simulink library "formationFlyingBlockset"  (R2016b)
settings: Solver=ode45  StartTime=0.0  StopTime=10.0  RelTol=1e-3  EnableMultiTasking=on
undefined symbols (not defined in the file or in its folder): adaptive, aircraftmask_ID, aircraftmask_navigationLaw, aircraftmask_originNED_ECEF_rrm, aircraftmask_p0_NED_m, aircraftmask_phithetapsi_trim, aircraftmask_wakevortexenabled, airkraftmask_displayLeader, DiscIntNeverNeededParam, Earth, fflib_degdegm2rrm, fflib_Hz2radps, fflib_rrm2degdegm, flat2lla, hinf, Klqr, lquadr, mask_ac, mask_ID, mpc, poleplacement, uavsim, washout, WGS84
undefined symbols (not defined in the file): aircraftmask_phithetapsi0, aircraftmask_pqr0, aircraftmask_uvw0, innerloop, outerloop, tatestos
libraries: formationFlyingBlockset x59, aerolibtransform2 x42, simulink_extras x27, dspsrcs4 x11, aerolibutil x5, uavsimBlockset_UAV3DInterface x4, uavsimBlockset_ServoHS55 x4, uavsimBlockset_VectorNorm x3, uavsimBlockset_UAV3DVisualization x3, uavsimBlockset_AugmentWind x3, stringquartett x2, Parrot_DCAS_lib x2
(part 5 of 5)

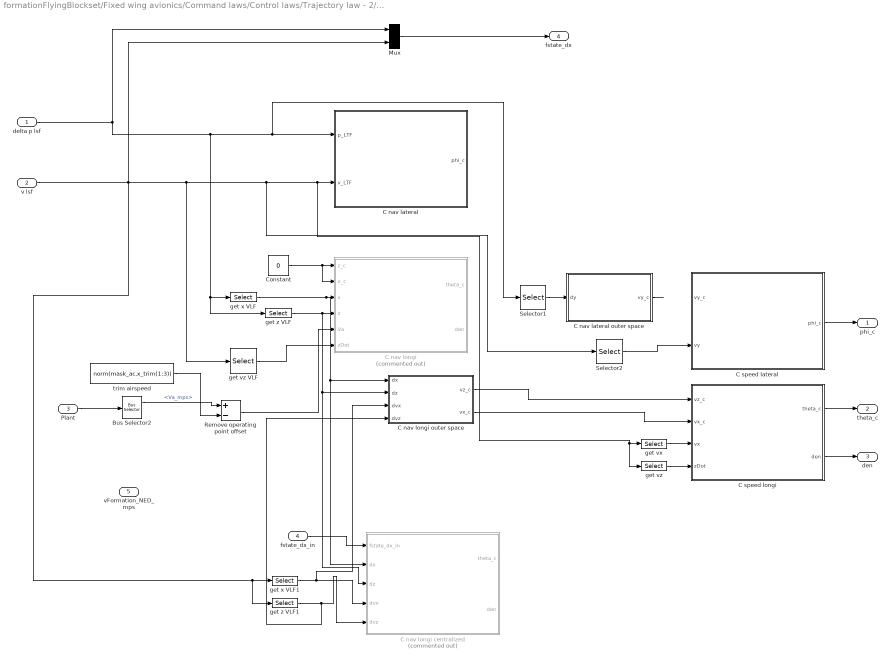
== system formationFlyingBlockset/Fixed wing avionics/Command laws/Control laws/Trajectory law - 2/Leader following laws/LQR nav loops ==
  delta p lsf : Inport
  v lsf : Inport  Port=2
  Plant : Inport  Port=3  OutDataTypeStr=Bus: StateBus
  fstate_dx_in : Inport  Port=4
  vFormation_NED_mps : Inport  Port=5
  Bus Selector2 : BusSelector  OutputSignals=Va_mps,v_ned_mps
  C nav lateral : Subsystem
  C nav lateral outer space : Subsystem
  C nav longi : Subsystem  Commented=on
  C nav longi centralized : Subsystem  Commented=on
  C nav longi outer space : Subsystem
  C speed lateral : Subsystem
  C speed longi : Subsystem
  Constant : Constant  Value=0
  Mux : Mux  Inputs=2
  Remove operating point offset : Sum  Inputs=+-
  Selector1 : Selector  InputPortWidth=3  IndexOptions=Index vector (dialog)  Indices=2  OutputSizes=1
  Selector2 : Selector  InputPortWidth=3  IndexOptions=Index vector (dialog)  Indices=2  OutputSizes=1
  get vx : Selector  InputPortWidth=3  IndexOptions=Index vector (dialog)  Indices=1  OutputSizes=1
  get vz : Selector  InputPortWidth=3  IndexOptions=Index vector (dialog)  Indices=3  OutputSizes=1
  get vz VLF : Selector  InputPortWidth=3  IndexOptions=Index vector (dialog)  Indices=3  OutputSizes=1
  get x VLF : Selector  InputPortWidth=3  IndexOptions=Index vector (dialog)  Indices=1  OutputSizes=1
  get x VLF1 : Selector  InputPortWidth=3  IndexOptions=Index vector (dialog)  Indices=1  OutputSizes=1
  get z VLF : Selector  InputPortWidth=3  IndexOptions=Index vector (dialog)  Indices=3  OutputSizes=1
  get z VLF1 : Selector  InputPortWidth=3  IndexOptions=Index vector (dialog)  Indices=3  OutputSizes=1
  trim airspeed : Constant  Value=norm(mask_ac.x_trim(1:3))
  phi_c : Outport  PortDimensions=1
  theta_c : Outport  Port=2  PortDimensions=1
  den : Outport  Port=3  PortDimensions=1
  fstate_dx : Outport  Port=4
  wires:
  C speed lateral/1(phi_c) -> phi_c/1
  v lsf/1 -> Mux/2, get vz VLF/1, C nav lateral/2(v_LTF), get vx/1, get vz/1, Selector2/1, get x VLF1/1, get z VLF1/1
  Selector2/1 -> C speed lateral/2(vy)
  C nav lateral outer space/1(vy_c) -> ?
  Selector1/1 -> C nav lateral outer space/1(dy)
  get z VLF1/1 -> C nav longi centralized/5(dvz), C nav longi outer space/4(dvz)
  C nav longi outer space/2(vx_c) -> C speed longi/2(vx_c)
  C nav longi outer space/1(vz_c) -> C speed longi/1(vz_c)
  get vz/1 -> C speed longi/4(zDot)
  get vx/1 -> C speed longi/3(vx)
  get x VLF1/1 -> C nav longi centralized/4(dvx), C nav longi outer space/3(dvx)
  delta p lsf/1 -> Mux/1, get z VLF/1, get x VLF/1, C nav lateral/1(p_LTF), Selector1/1
  Constant/1 -> C nav longi/2(x_c), C nav longi/1(z_c)
  get z VLF/1 -> C nav longi/4(z), C nav longi centralized/3(dz), C nav longi outer space/2(dz)
  get x VLF/1 -> C nav longi/3(x), C nav longi centralized/2(dx), C nav longi outer space/1(dx)
  Remove operating point offset/1 -> C nav longi/5(Va)
  get vz VLF/1 -> C nav longi/6(zDot)
  C speed longi/1(theta_c) -> theta_c/1
  C speed longi/2(den) -> den/1
  Plant/1 -> Bus Selector2/1
  Bus Selector2/1 -> Remove operating point offset/1  "<Va_mps>"
  trim airspeed/1 -> Remove operating point offset/2
  fstate_dx_in/1 -> C nav longi centralized/1(fstate_dx_in)
  Mux/1 -> fstate_dx/1

== system formationFlyingBlockset/Fixed wing avionics/Command laws/Control laws/Trajectory law - 2/Leader following laws/Manual tuning SISO outer loops ==
  "\tIntegrator reset signal" : Inport
  v lsf : Inport  Port=2
  p lsf : Inport  Port=3
  Trigger : TriggerPort  TriggerType=either  VariantControl=Variant  PortDimensions=1
  Altitude controller : Subsystem
  Lateral trajectory deviation controller : Subsystem
  Longitudinal trajectory deviation controller : Subsystem
  theta_c : Outport
  phi_c : Outport  Port=2
  delta_en : Outport  Port=3
  wires:
  Altitude controller/1(theta_c) -> theta_c/1
  "\tIntegrator reset signal"/1 -> Longitudinal trajectory deviation controller/3(Integrator Reset), Altitude controller/1(Integrator Reset)
  Longitudinal trajectory deviation controller/1(delta_en) -> delta_en/1
  Lateral trajectory deviation controller/1(phi_c) -> phi_c/1
  p lsf/1 -> Altitude controller/3(p lsf), Longitudinal trajectory deviation controller/1(p_ERRF), Lateral trajectory deviation controller/1(p_ERRF)
  v lsf/1 -> Lateral trajectory deviation controller/2(v_ERRF), Altitude controller/2(v lsf), Longitudinal trajectory deviation controller/2(v_ERRF)

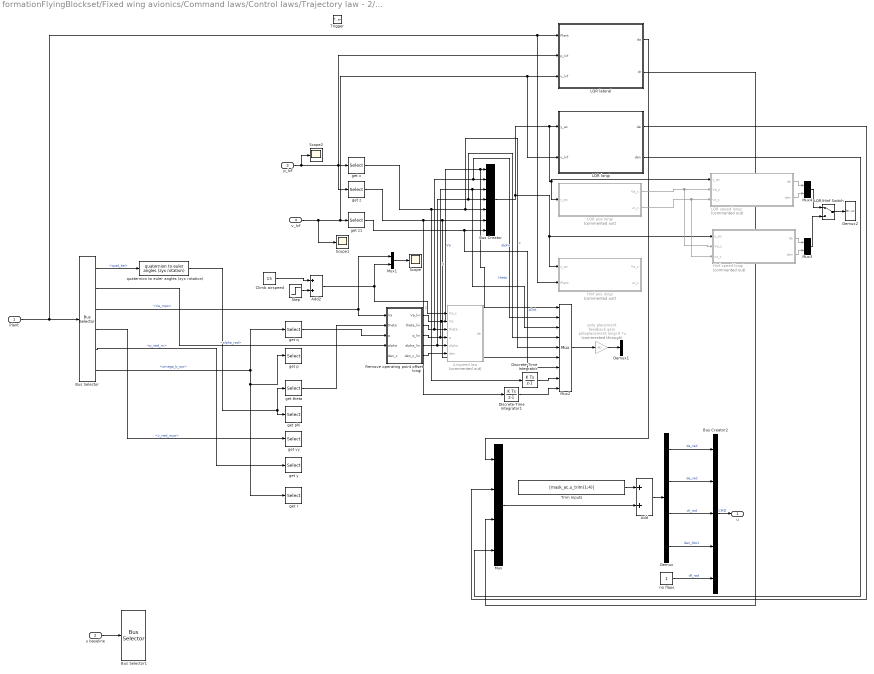
== system formationFlyingBlockset/Fixed wing avionics/Command laws/Control laws/Trajectory law - 2/Leader following laws/Non-nested laws ==
  Plant : Inport  OutDataTypeStr=Bus: StateBus
  u baseline : Inport  Port=2  OutDataTypeStr=Bus: CMD
  p_lvf : Inport  Port=3
  v_lvf : Inport  Port=4
  Trigger : TriggerPort  TriggerType=either  VariantControl=Variant  PortDimensions=1
  Add : Sum
  Add2 : Sum
  Airspeed law : Subsystem  Commented=on
  Bus Creator : BusCreator  Inputs='Va','theta','q','alpha','x','z','zDot'
  Bus Creator2 : BusCreator  Inputs=5  OutDataTypeStr=Bus: CMD  NonVirtualBus=on
  Bus Selector : BusSelector  OutputSignals=quat_be,alpha_rad,Va_mps,v_ned_mps,p_ned_m,omega_b_rps
  Bus Selector1 : BusSelector  OutputSignals=da_rad,de_rad,den_0to1
  Climb airspeed : Constant  Value=15
  Demux : Demux
  Demux1 : Demux  Outputs=2
  Demux2 : Demux  Outputs=2
  Discrete-Time Integrator : DiscreteIntegrator  InitialConditionSetting=State (most efficient)  SampleTime=-1  ICPrevOutput=DiscIntNeverNeededParam  ICPrevScaledInput=DiscIntNeverNeededParam
  Discrete-Time Integrator1 : DiscreteIntegrator  InitialConditionSetting=State (most efficient)  SampleTime=-1  ICPrevOutput=DiscIntNeverNeededParam  ICPrevScaledInput=DiscIntNeverNeededParam
  Hinf pos longi : Subsystem  Commented=on
  Hinf speed longi : Subsystem  Commented=on
  LQR lateral : Subsystem
  LQR longi : Subsystem
  LQR pos longi : Subsystem  Commented=on
  LQR speed longi : Subsystem  Commented=on
  LQR/Hinf Switch : ManualSwitch
  Mux : Mux
  Mux1 : Mux  Inputs=2
  Mux2 : Mux  Inputs=9
  Mux3 : Mux  Inputs=2
  Mux4 : Mux  Inputs=2
  Remove operating point offset longi : Subsystem
  Scope : Scope
  Scope1 : Scope
  Scope2 : Scope
  Step : Step  Time=12  After=5
  Trim Inputs : Constant  Value=[mask_ac.u_trim(1:4)]
  get p : Selector  InputPortWidth=3  IndexOptions=Index vector (dialog)  Indices=[1]  OutputSizes=1
  get phi : Selector  InputPortWidth=3  IndexOptions=Index vector (dialog)  Indices=[1]  OutputSizes=1
  get q : Selector  InputPortWidth=3  IndexOptions=Index vector (dialog)  Indices=2  OutputSizes=1
  get r : Selector  InputPortWidth=3  IndexOptions=Index vector (dialog)  Indices=3  OutputSizes=1
  get theta : Selector  InputPortWidth=3  IndexOptions=Index vector (dialog)  Indices=2  OutputSizes=1
  get vy : Selector  InputPortWidth=3  IndexOptions=Index vector (dialog)  Indices=2  OutputSizes=1
  get x : Selector  InputPortWidth=3  IndexOptions=Index vector (dialog)  Indices=1  OutputSizes=1
  get y : Selector  InputPortWidth=3  IndexOptions=Index vector (dialog)  Indices=2  OutputSizes=1
  get z : Selector  InputPortWidth=3  IndexOptions=Index vector (dialog)  Indices=3  OutputSizes=1
  get z1 : Selector  InputPortWidth=3  IndexOptions=Index vector (dialog)  Indices=3  OutputSizes=1
  no flaps : Constant
  pole placement feedback gain : Gain  Commented=through  Gain=poleplacement.longi.K  Multiplication=Matrix(K*u)
  quaternion to euler angles (zyx rotation) : formationFlyingBlockset/quaternion to euler  angles (zyx rotation)
  u : Outport  OutDataTypeStr=Bus: CMD
  wires:
  Bus Creator2/1 -> u/1  "CMD"
  Demux/3 -> Bus Creator2/3  "dr_rad"
  Demux/4 -> Bus Creator2/4  "den_0to1"
  Demux/1 -> Bus Creator2/1  "da_rad"
  Demux/2 -> Bus Creator2/2  "de_rad"
  Trim Inputs/1 -> Add/1
  Add/1 -> Demux/1
  Mux/1 -> Add/2
  no flaps/1 -> Bus Creator2/5  "df_rad"
  quaternion to euler angles (zyx rotation)/1 -> get phi/1, get theta/1
  Bus Selector/2 -> Remove operating point offset longi/4(alpha)  "<alpha_rad>"
  Bus Selector/3 -> Remove operating point offset longi/1(Va), Mux1/1  "<Va_mps>"
  Climb airspeed/1 -> Add2/1
  Step/1 -> Add2/2
  get theta/1 -> Remove operating point offset longi/2(theta)
  Bus Selector/4 -> get vy/1  "<v_ned_mps>"
  Bus Selector/5 -> get y/1  "<p_ned_m>"
  Bus Selector/6 -> get r/1, get p/1, get q/1  "<omega_b_rps>"
  get q/1 -> Remove operating point offset longi/3(q)
  u baseline/1 -> Bus Selector1/1
  Remove operating point offset longi/5(den_c_lin) -> Airspeed law/6(den)
  Add2/1 -> Airspeed law/1(Va_c), Mux1/2
  Mux1/1 -> Scope/1
  Bus Selector/1 -> quaternion to euler angles (zyx rotation)/1  "<quat_be>"
  Remove operating point offset longi/1(Va_lin) -> Mux2/1, Bus Creator/1, Airspeed law/2(Va)  "Va"
  get x/1 -> Discrete-Time Integrator/1, Mux2/5, Bus Creator/5  "x"
  get z/1 -> Discrete-Time Integrator1/1, Bus Creator/6, Mux2/6  "z"
  Remove operating point offset longi/2(theta_lin) -> Mux2/2, Bus Creator/2, Airspeed law/3(theta)  "theta"
  Remove operating point offset longi/3(q_lin) -> Mux2/3, Bus Creator/3, Airspeed law/4(q)  "q"
  Remove operating point offset longi/4(alpha_lin) -> Mux2/4, Bus Creator/4, Airspeed law/5(alpha)  "alpha"
  p_lvf/1 -> Scope2/1, LQR lateral/2(p_lvf), get z/1, get x/1
  v_lvf/1 -> Scope1/1, LQR longi/2(v_lvf), LQR lateral/3(v_lvf), get z1/1
  get z1/1 -> Mux2/7, Bus Creator/7  "zDot"
  Bus Creator/1 -> Hinf pos longi/1(y_ac), Hinf speed longi/1(y_ac), LQR pos longi/1(y_ac), LQR speed longi/1(y_ac), LQR longi/1(y_ac)
  LQR longi/1(de) -> Mux/2
  LQR longi/2(den) -> Mux/4
  Mux2/1 -> pole placement feedback gain/1
  pole placement feedback gain/1 -> Demux1/1
  Discrete-Time Integrator/1 -> Mux2/8
  Discrete-Time Integrator1/1 -> Mux2/9
  LQR lateral/1(da) -> Mux/1
  LQR lateral/2(dr) -> Mux/3
  Plant/1 -> Hinf pos longi/2(Plant), LQR lateral/1(Plant), Bus Selector/1
  LQR pos longi/1(Va_c) -> Hinf speed longi/2(Va_c), LQR speed longi/2(Va_c)
  LQR pos longi/2(vz_c) -> Hinf speed longi/3(vz_c), LQR speed longi/3(vz_c)
  LQR speed longi/2(den) -> Mux4/2
  LQR speed longi/1(de) -> Mux4/1
  Hinf speed longi/1(de) -> Mux3/1
  Hinf speed longi/2(den) -> Mux3/2
  Mux4/1 -> LQR/Hinf Switch/1
  Mux3/1 -> LQR/Hinf Switch/2
  LQR/Hinf Switch/1 -> Demux2/1

== system formationFlyingBlockset/Fixed wing avionics/Command laws/Control laws/Trajectory law - 2/Leader following laws/Hinf outer loops1/C PI dy ==
  p_LTF : Inport
  v_LTF : Inport  Port=2
  Add : Sum  Inputs=+-
  Discrete-Time Integrator1 : DiscreteIntegrator  SampleTime=-1  ICPrevOutput=DiscIntNeverNeededParam  ICPrevScaledInput=DiscIntNeverNeededParam
  Ky : Gain  Gain=uavsim.ap.control.Hinf_y.Ky  Multiplication=Matrix(K*u)
  Mux1 : Mux
  Selector : Selector  InputPortWidth=3  IndexOptions=Index vector (dialog)  Indices=2  OutputSizes=1
  Selector1 : Selector  InputPortWidth=3  IndexOptions=Index vector (dialog)  Indices=2  OutputSizes=1
  Step : Step  Time=12  After=0
  dy_c : Constant  Value=0
  phi_c : Outport
  wires:
  Ky/1 -> phi_c/1
  dy_c/1 -> Mux1/1
  Selector/1 -> Add/1  "e"
  Step/1 -> Add/2
  Selector1/1 -> Mux1/4
  Discrete-Time Integrator1/1 -> Mux1/2
  Add/1 -> Discrete-Time Integrator1/1, Mux1/3
  Mux1/1 -> Ky/1
  v_LTF/1 -> Selector1/1
  p_LTF/1 -> Selector/1

== system formationFlyingBlockset/Fixed wing avionics/Command laws/Control laws/Trajectory law - 2/Leader following laws/Hinf outer loops1/C nav ==
  z_c : Inport
  x_c : Inport  Port=2
  x : Inport  Port=3
  z : Inport  Port=4
  Va : Inport  Port=5
  zDot : Inport  Port=6
  Add1 : Sum  Inputs=-+
  Demux : Demux  Outputs=2
  Discrete-Time Integrator : DiscreteIntegrator  gainval=10  InitialConditionSetting=State (most efficient)  SampleTime=-1  ICPrevOutput=DiscIntNeverNeededParam  ICPrevScaledInput=DiscIntNeverNeededParam
  Klongi_nav : Gain  Gain=uavsim.ap.control.Hinf_longi.Klongi_nav  Multiplication=Matrix(K*u)
  Mux1 : Mux
  Mux2 : Mux  Inputs=2
  Mux3 : Mux  Inputs=2
  Scope : Scope
  Scope1 : Scope
  theta_c : Outport
  den : Outport  Port=2
  wires:
  zDot/1 -> Mux1/4
  Demux/2 -> den/1
  Demux/1 -> theta_c/1
  Va/1 -> Mux1/3
  Mux3/1 -> Add1/2
  Mux2/1 -> Add1/1
  z/1 -> Mux3/2
  x/1 -> Mux3/1
  z_c/1 -> Mux2/2
  x_c/1 -> Mux2/1
  Discrete-Time Integrator/1 -> Mux1/1, Scope/1
  Add1/1 -> Mux1/2, Scope1/1, Discrete-Time Integrator/1  "e"
  Mux1/1 -> Klongi_nav/1
  Klongi_nav/1 -> Demux/1

== system formationFlyingBlockset/Fixed wing avionics/Command laws/Control laws/Trajectory law - 2/Leader following laws/LQR nav loops/C nav lateral ==
  p_LTF : Inport
  v_LTF : Inport  Port=2
  Add : Sum  Inputs=+-
  Discrete-Time Integrator1 : DiscreteIntegrator  SampleTime=-1  ICPrevOutput=DiscIntNeverNeededParam  ICPrevScaledInput=DiscIntNeverNeededParam
  Ky : Gain  Gain=uavsim.ap.control.lquadr.latnav.K  Multiplication=Matrix(K*u)
  Mux1 : Mux  Inputs=3
  Selector : Selector  InputPortWidth=3  IndexOptions=Index vector (dialog)  Indices=2  OutputSizes=1
  Selector1 : Selector  InputPortWidth=3  IndexOptions=Index vector (dialog)  Indices=2  OutputSizes=1
  Step : Step  Time=12  After=0
  phi_c : Outport
  wires:
  p_LTF/1 -> Selector/1
  v_LTF/1 -> Selector1/1
  Mux1/1 -> Ky/1
  Add/1 -> Discrete-Time Integrator1/1, Mux1/1
  Discrete-Time Integrator1/1 -> Mux1/3
  Selector1/1 -> Mux1/2
  Step/1 -> Add/2
  Selector/1 -> Add/1  "e"
  Ky/1 -> phi_c/1

== system formationFlyingBlockset/Fixed wing avionics/Command laws/Control laws/Trajectory law - 2/Leader following laws/LQR nav loops/C nav lateral outer space ==
  dy : Inport
  Gain : Gain  Gain=-0.5
  Scope1 : Scope  NumInputPorts=2
  Scope2 : Scope  NumInputPorts=2
  vy_c : Outport
  wires:
  dy/1 -> Scope2/1, Gain/1
  Gain/1 -> vy_c/1, Scope1/1

== system formationFlyingBlockset/Fixed wing avionics/Command laws/Control laws/Trajectory law - 2/Leader following laws/LQR nav loops/C nav longi ==
  z_c : Inport
  x_c : Inport  Port=2
  x : Inport  Port=3
  z : Inport  Port=4
  Va : Inport  Port=5
  zDot : Inport  Port=6
  Add1 : Sum  Inputs=-+
  Demux : Demux  Outputs=2
  Discrete-Time Integrator : DiscreteIntegrator  gainval=1  InitialConditionSetting=State (most efficient)  SampleTime=-1  ICPrevOutput=DiscIntNeverNeededParam  ICPrevScaledInput=DiscIntNeverNeededParam
  Gain : Gain  Gain=uavsim.ap.control.lquadr.longinav.K  Multiplication=Matrix(K*u)
  Gain1 : Gain  Gain=evalin('base', ['longinav_decentralized.K' num2str(aircraftmask_ID)])  Multiplication=Matrix(K*u)
  Gain2 : Gain  Gain=-1
  Gain3 : Gain  Gain=-1
  Gain4 : Gain  Gain=-1
  Mux1 : Mux
  Mux{2..5} (4 alike) : Mux  Inputs=2
  Mux6 : Mux  Inputs=3
  Scope : Scope
  Scope1 : Scope
  Scope2 : Scope  NumInputPorts=2
  theta_c : Outport
  den : Outport  Port=2
  wires:
  Gain4/1 -> Mux6/3
  Gain3/1 -> Mux6/2
  Gain2/1 -> Mux6/1
  zDot/1 -> Mux1/2, Gain4/1
  Mux6/1 -> Gain1/1
  Gain1/1 -> Demux/1
  Add1/1 -> Discrete-Time Integrator/1, Mux1/3, Scope1/1, Gain2/1  "e"
  Discrete-Time Integrator/1 -> Mux1/4, Scope/1
  x_c/1 -> Mux4/1, Mux2/1
  z_c/1 -> Mux5/1, Mux2/2
  x/1 -> Mux4/2, Mux3/1
  z/1 -> Mux5/2, Mux3/2
  Mux2/1 -> Add1/1
  Mux3/1 -> Add1/2
  Va/1 -> Mux1/1, Gain3/1
  Demux/2 -> theta_c/1
  Demux/1 -> den/1
  Mux1/1 -> Gain/1
  Mux4/1 -> Scope2/1  "x"
  Mux5/1 -> Scope2/2  "z"

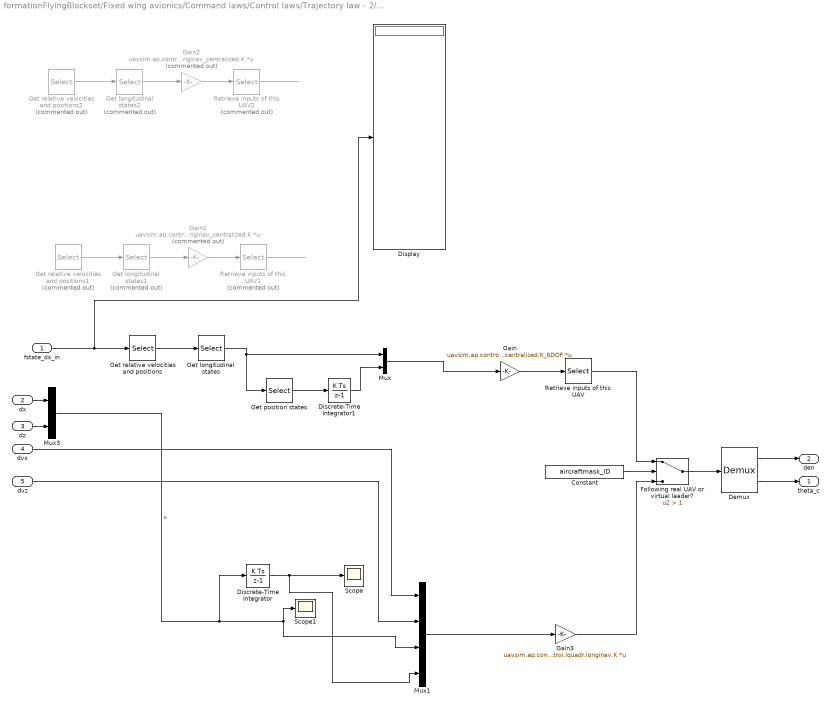
== system formationFlyingBlockset/Fixed wing avionics/Command laws/Control laws/Trajectory law - 2/Leader following laws/LQR nav loops/C nav longi centralized ==
  fstate_dx_in : Inport
  dx : Inport  Port=2
  dz : Inport  Port=3
  dvx : Inport  Port=4
  dvz : Inport  Port=5
  Constant : Constant  Value=aircraftmask_ID
  Demux : Demux  Outputs=2
  Discrete-Time Integrator : DiscreteIntegrator  gainval=1  InitialConditionSetting=State (most efficient)  SampleTime=-1  ICPrevOutput=DiscIntNeverNeededParam  ICPrevScaledInput=DiscIntNeverNeededParam
  Discrete-Time Integrator1 : DiscreteIntegrator  InitialConditionSetting=State (most efficient)  SampleTime=-1  ICPrevOutput=DiscIntNeverNeededParam  ICPrevScaledInput=DiscIntNeverNeededParam
  Display : Display
  Following real UAV or virtual leader? : Switch  Criteria=u2 > Threshold  Threshold=1
  Gain : Gain  Gain=uavsim.ap.control.lquadr.longinav_centralized.K_6DOF  Multiplication=Matrix(K*u)
  Gain1 : Gain  Commented=on  Gain=uavsim.ap.control.lquadr.longinav_centralized.K  Multiplication=Matrix(K*u)
  Gain2 : Gain  Commented=on  Gain=uavsim.ap.control.lquadr.longinav_centralized.K  Multiplication=Matrix(K*u)
  Gain3 : Gain  Gain=uavsim.ap.control.lquadr.longinav.K  Multiplication=Matrix(K*u)
  Get longitudinal states : Selector  InputPortWidth=12  IndexOptions=Index vector (dialog)  Indices=[1 3 4 6 7 9 10 12]  OutputSizes=1
  Get longitudinal states1 : Selector  Commented=on  InputPortWidth=12  IndexOptions=Index vector (dialog)  Indices=[4 6 1 3 10 12 7 9]  OutputSizes=1
  Get longitudinal states2 : Selector  Commented=on  InputPortWidth=6  IndexOptions=Index vector (dialog)  Indices=[1 3 4 6]  OutputSizes=1
  Get position states : Selector  InputPortWidth=8  IndexOptions=Index vector (dialog)  Indices=[1 2 5 6]  OutputSizes=1
  Get relative velocities and positions : Selector  InputPortWidth=18  IndexOptions=Index vector (dialog)  Indices=7:18  OutputSizes=1
  Get relative velocities and positions1 : Selector  Commented=on  InputPortWidth=18  IndexOptions=Index vector (dialog)  Indices=7:18  OutputSizes=1
  Get relative velocities and positions2 : Selector  Commented=on  InputPortWidth=12  IndexOptions=Index vector (dialog)  Indices=7:12  OutputSizes=1
  Mux : Mux  Inputs=2
  Mux1 : Mux
  Mux3 : Mux  Inputs=2
  Retrieve inputs of this UAV : Selector  InputPortWidth=6  IndexOptions=Index vector (dialog)  Indices=[(aircraftmask_ID)*2 - 1 : (aircraftmask_ID)*2 ]  OutputSizes=1
  Retrieve inputs of this UAV1 : Selector  Commented=on  InputPortWidth=6  IndexOptions=Index vector (dialog)  Indices=[(aircraftmask_ID)*2 - 1 : (aircraftmask_ID)*2 ]  OutputSizes=1
  Retrieve inputs of this UAV2 : Selector  Commented=on  InputPortWidth=4  IndexOptions=Index vector (dialog)  Indices=[(aircraftmask_ID)*2 - 1 : (aircraftmask_ID)*2 ]  OutputSizes=1
  Scope : Scope
  Scope1 : Scope
  theta_c : Outport
  den : Outport  Port=2
  wires:
  Discrete-Time Integrator1/1 -> Mux/2
  Get position states/1 -> Discrete-Time Integrator1/1
  Get longitudinal states/1 -> Get position states/1, Mux/1
  Following real UAV or virtual leader?/1 -> Demux/1
  Constant/1 -> Following real UAV or virtual leader?/2
  dvz/1 -> Mux1/2
  Gain3/1 -> Following real UAV or virtual leader?/3
  Mux3/1 -> Discrete-Time Integrator/1, Mux1/3, Scope1/1  "e"
  Discrete-Time Integrator/1 -> Mux1/4, Scope/1
  dvx/1 -> Mux1/1
  Mux1/1 -> Gain3/1
  dx/1 -> Mux3/1
  dz/1 -> Mux3/2
  Gain2/1 -> Retrieve inputs of this UAV2/1
  Get relative velocities and positions2/1 -> Get longitudinal states2/1
  Get longitudinal states2/1 -> Gain2/1
  Retrieve inputs of this UAV2/1 -> ?
  Gain1/1 -> Retrieve inputs of this UAV1/1
  Get relative velocities and positions1/1 -> Get longitudinal states1/1
  Get longitudinal states1/1 -> Gain1/1
  Retrieve inputs of this UAV1/1 -> ?
  Demux/1 -> den/1
  Demux/2 -> theta_c/1
  Gain/1 -> Retrieve inputs of this UAV/1
  fstate_dx_in/1 -> Get relative velocities and positions/1, Display/1
  Get relative velocities and positions/1 -> Get longitudinal states/1
  Mux/1 -> Gain/1
  Retrieve inputs of this UAV/1 -> Following real UAV or virtual leader?/1

== system formationFlyingBlockset/Fixed wing avionics/Command laws/Control laws/Trajectory law - 2/Leader following laws/LQR nav loops/C nav longi outer space ==
  dx : Inport
  dz : Inport  Port=2
  dvx : Inport  Port=3
  dvz : Inport  Port=4
  Scope1 : Scope  NumInputPorts=2
  Scope2 : Scope  NumInputPorts=2
  pos control discrete : stringquartett/pos control discrete
  pos control discrete1 : stringquartett/pos control discrete
  vz_c : Outport
  vx_c : Outport  Port=2
  wires:
  dvz/1 -> pos control discrete1/2
  dvx/1 -> pos control discrete/2
  pos control discrete1/1 -> vz_c/1
  pos control discrete/1 -> Scope1/1, vx_c/1
  dz/1 -> Scope2/2, pos control discrete1/1  "dz"
  dx/1 -> Scope2/1, pos control discrete/1  "dx"

== system formationFlyingBlockset/Fixed wing avionics/Command laws/Control laws/Trajectory law - 2/Leader following laws/LQR nav loops/C speed lateral ==
  vy_c : Inport
  vy : Inport  Port=2
  Add1 : Sum  Inputs=-+
  Discrete-Time Integrator : DiscreteIntegrator  gainval=1  InitialConditionSetting=State (most efficient)  SampleTime=-1  ICPrevOutput=DiscIntNeverNeededParam  ICPrevScaledInput=DiscIntNeverNeededParam
  Gain : Gain  Gain=uavsim.ap.control.lquadr.lateralspeed.K  Multiplication=Matrix(K*u)
  Mux1 : Mux  Inputs=2
  Mux4 : Mux  Inputs=2
  Scope : Scope
  Scope1 : Scope
  Scope2 : Scope
  phi_c : Outport
  wires:
  Mux1/1 -> Gain/1
  Add1/1 -> Discrete-Time Integrator/1, Mux1/1, Scope1/1  "e"
  Discrete-Time Integrator/1 -> Mux1/2, Scope/1
  vy_c/1 -> Add1/1, Mux4/1
  Gain/1 -> phi_c/1
  vy/1 -> Mux4/2, Add1/2
  Mux4/1 -> Scope2/1

== system formationFlyingBlockset/Fixed wing avionics/Command laws/Control laws/Trajectory law - 2/Leader following laws/LQR nav loops/C speed longi ==
  vz_c : Inport
  vx_c : Inport  Port=2
  vx : Inport  Port=3
  zDot : Inport  Port=4
  Add1 : Sum  Inputs=-+
  Demux : Demux  Outputs=2
  Discrete-Time Integrator : DiscreteIntegrator  gainval=1  InitialConditionSetting=State (most efficient)  SampleTime=-1  ICPrevOutput=DiscIntNeverNeededParam  ICPrevScaledInput=DiscIntNeverNeededParam
  Gain : Gain  Gain=uavsim.ap.control.lquadr.longispeed.K  Multiplication=Matrix(K*u)
  Mux{1..4} (4 alike) : Mux  Inputs=2
  Scope : Scope
  Scope1 : Scope
  Scope2 : Scope
  theta_c : Outport
  den : Outport  Port=2
  wires:
  Gain/1 -> Demux/1
  Mux4/1 -> Scope2/1
  Mux3/1 -> Add1/2, Mux4/2
  zDot/1 -> Mux3/2
  vx/1 -> Mux3/1
  Mux1/1 -> Gain/1
  Demux/1 -> den/1
  Demux/2 -> theta_c/1
  Mux2/1 -> Add1/1, Mux4/1
  vz_c/1 -> Mux2/2
  vx_c/1 -> Mux2/1
  Discrete-Time Integrator/1 -> Scope/1, Mux1/2
  Add1/1 -> Scope1/1, Mux1/1, Discrete-Time Integrator/1  "e"

== system formationFlyingBlockset/Fixed wing avionics/Command laws/Control laws/Trajectory law - 2/Leader following laws/Manual tuning SISO outer loops/Altitude controller ==
  Integrator Reset : Inport
  v lsf : Inport  Port=2
  p lsf : Inport  Port=3
  Discrete-Time Integrator : DiscreteIntegrator  ExternalReset=either  SampleTime=-1  ICPrevOutput=DiscIntNeverNeededParam  ICPrevScaledInput=DiscIntNeverNeededParam
  Gain : Gain  Gain=[0 0.3 0.1]  Multiplication=Matrix(K*u)
  Mux : Mux  Inputs=3
  Scope : Scope  NumInputPorts=2
  get vz : Selector  InputPortWidth=3  IndexOptions=Index vector (dialog)  Indices=3  OutputSizes=1
  get z : Selector  InputPortWidth=3  IndexOptions=Index vector (dialog)  Indices=3  OutputSizes=1
  theta_c : Outport
  wires:
  Integrator Reset/1 -> Discrete-Time Integrator/2
  p lsf/1 -> get z/1  "z"
  Discrete-Time Integrator/1 -> Mux/1
  Mux/1 -> Gain/1
  Gain/1 -> theta_c/1
  v lsf/1 -> get vz/1  "vz"
  get z/1 -> Scope/1, Mux/2, Discrete-Time Integrator/1
  get vz/1 -> Scope/2, Mux/3

== system formationFlyingBlockset/Fixed wing avionics/Command laws/Control laws/Trajectory law - 2/Leader following laws/Manual tuning SISO outer loops/Lateral trajectory deviation controller ==
  p_ERRF : Inport
  v_ERRF : Inport  Port=2
  Demux : Demux  Outputs=3
  Demux1 : Demux  Outputs=3
  Gain : Gain  Gain=[-0.2 -0.2]  Multiplication=Matrix(K*u)
  Mux1 : Mux  Inputs=2
  dx : Scope
  dy : Scope
  dz : Scope
  vx : Scope
  vy : Scope
  vz : Scope
  phi_c : Outport
  wires:
  v_ERRF/1 -> Demux1/1
  p_ERRF/1 -> Demux/1
  Mux1/1 -> Gain/1
  Demux1/3 -> vz/1
  Demux1/1 -> vx/1
  Demux1/2 -> vy/1, Mux1/2
  Demux/3 -> dz/1
  Demux/1 -> dx/1
  Demux/2 -> dy/1, Mux1/1
  Gain/1 -> phi_c/1

== system formationFlyingBlockset/Fixed wing avionics/Command laws/Control laws/Trajectory law - 2/Leader following laws/Manual tuning SISO outer loops/Longitudinal trajectory deviation controller ==
  p_ERRF : Inport
  v_ERRF : Inport  Port=2
  Integrator Reset : Inport  Port=3
  Discrete-Time Integrator : DiscreteIntegrator  ExternalReset=either  SampleTime=-1  ICPrevOutput=DiscIntNeverNeededParam  ICPrevScaledInput=DiscIntNeverNeededParam
  Gain : Gain  Gain=[-0.05 -0.5 -0.2]  Multiplication=Matrix(K*u)
  Mux1 : Mux  Inputs=3
  get vx : Selector  InputPortWidth=3  IndexOptions=Index vector (dialog)  Indices=1  OutputSizes=1
  get x : Selector  InputPortWidth=3  IndexOptions=Index vector (dialog)  Indices=1  OutputSizes=1
  int(px) : Scope
  px : Scope
  vx : Scope
  delta_en : Outport
  wires:
  Integrator Reset/1 -> Discrete-Time Integrator/2
  Discrete-Time Integrator/1 -> int(px)/1, Mux1/1
  get x/1 -> Mux1/2, Discrete-Time Integrator/1, px/1
  get vx/1 -> Mux1/3, vx/1
  Gain/1 -> delta_en/1
  v_ERRF/1 -> get vx/1
  Mux1/1 -> Gain/1
  p_ERRF/1 -> get x/1

== system formationFlyingBlockset/Fixed wing avionics/Command laws/Control laws/Trajectory law - 2/Leader following laws/Non-nested laws/Airspeed law ==
  Va_c : Inport  PortDimensions=1
  Va : Inport  Port=2  PortDimensions=1
  theta : Inport  Port=3  PortDimensions=1
  q : Inport  Port=4  PortDimensions=1
  alpha : Inport  Port=5  PortDimensions=1
  den : Inport  Port=6  PortDimensions=1
  Add1 : Sum  Inputs=-+
  Add2 : Sum
  Discrete-Time Integrator : DiscreteIntegrator  SampleTime=-1  ICPrevOutput=DiscIntNeverNeededParam  ICPrevScaledInput=DiscIntNeverNeededParam
  K_airspeed : Gain  Gain=uavsim.ap.control.Hinf.Va.K_airspeed  Multiplication=Matrix(K*u)
  K_throttle : Gain  Gain=uavsim.ap.control.Hinf.Va.K_throttle  Multiplication=Matrix(K*u)
  Mux1 : Mux  Inputs=5
  de : Outport
  wires:
  Mux1/1 -> K_airspeed/1
  Va/1 -> Add1/2
  Va_c/1 -> Add1/1
  Add1/1 -> Discrete-Time Integrator/1, Mux1/1  "e"
  K_airspeed/1 -> Add2/1  "de"
  q/1 -> Mux1/4
  alpha/1 -> Mux1/5
  theta/1 -> Mux1/3
  Discrete-Time Integrator/1 -> Mux1/2
  den/1 -> K_throttle/1
  K_throttle/1 -> Add2/2  "de"
  Add2/1 -> de/1

== system formationFlyingBlockset/Fixed wing avionics/Command laws/Control laws/Trajectory law - 2/Leader following laws/Non-nested laws/Hinf pos longi ==
  y_ac : Inport
  Plant : Inport  Port=2  OutDataTypeStr=Bus: StateBus
  Bus Selector : BusSelector  OutputSignals=x,z
  Bus Selector1 : BusSelector  OutputSignals=v_ned_mps
  Discrete-Time Integrator1 : DiscreteIntegrator  InitialConditionSetting=State (most efficient)  SampleTime=-1  ICPrevOutput=DiscIntNeverNeededParam  ICPrevScaledInput=DiscIntNeverNeededParam
  Gain : Gain
  K_pos_x : Gain  Gain=hinf.longi.K_pos_x  Multiplication=Matrix(K*u)
  K_pos_z : Gain  Gain=hinf.longi.K_pos_z  Multiplication=Matrix(K*u)
  Mux2 : Mux  Inputs=2
  Mux4 : Mux  Inputs=2
  Mux5 : Mux  Inputs=2
  Scope7 : Scope
  Selector : Selector  InputPortWidth=3  IndexOptions=Index vector (dialog)  Indices=3  OutputSizes=1
  Selector1 : Selector  InputPortWidth=4  IndexOptions=Index vector (dialog)  Indices=[1 3]  OutputSizes=1
  Selector2 : Selector  InputPortWidth=4  IndexOptions=Index vector (dialog)  Indices=[2 4]  OutputSizes=1
  Step : Step  Time=10
  Va_c : Outport
  vz_c : Outport  Port=2
  wires:
  Selector/1 -> Gain/1, Mux5/2
  Bus Selector/2 -> Mux2/2  "<z>"
  Mux5/1 -> Scope7/1
  Bus Selector1/1 -> Selector/1  "<v_ned_mps>"
  Plant/1 -> Bus Selector1/1
  K_pos_z/1 -> ?
  K_pos_x/1 -> Va_c/1
  y_ac/1 -> Bus Selector/1
  Bus Selector/1 -> Mux2/1  "<x>"
  Mux2/1 -> Mux4/2, Discrete-Time Integrator1/1
  Discrete-Time Integrator1/1 -> Mux4/1
  Mux4/1 -> Selector2/1, Selector1/1
  Selector2/1 -> K_pos_z/1
  Selector1/1 -> K_pos_x/1
  Step/1 -> vz_c/1

== system formationFlyingBlockset/Fixed wing avionics/Command laws/Control laws/Trajectory law - 2/Leader following laws/Non-nested laws/Hinf speed longi ==
  y_ac : Inport
  Va_c : Inport  Port=2
  vz_c : Inport  Port=3
  Add2 : Sum  Inputs=-+
  Bus Selector : BusSelector  OutputSignals=Va,zDot,alpha,q,theta
  Demux : Demux  Outputs=2
  Demux2 : Demux  Outputs=2
  Discrete-Time Integrator : DiscreteIntegrator  InitialConditionSetting=State (most efficient)  SampleTime=-1  ICPrevOutput=DiscIntNeverNeededParam  ICPrevScaledInput=DiscIntNeverNeededParam
  K_speed : Gain  Gain=hinf.longi.K_speed  Multiplication=Matrix(K*u)
  LQR or Hinf? : ManualSwitch
  Mux{,1..2,4} (4 alike) : Mux  Inputs=2
  Mux3 : Mux
  Scope{,1..4,6} (6 alike) : Scope
  de : Outport
  den : Outport  Port=2
  wires:
  y_ac/1 -> Bus Selector/1
  Mux3/1 -> Scope/1, K_speed/1
  Add2/1 -> Mux3/3, Discrete-Time Integrator/1, Scope3/1
  K_speed/1 -> Demux2/1
  Mux1/1 -> Mux3/4, Scope4/1  "q, alpha"
  Demux2/1 -> Mux/1, Scope1/1  "den"
  Demux2/2 -> Mux/2, Scope2/1  "de"
  Bus Selector/4 -> Mux1/2  "<q>"
  Bus Selector/1 -> Mux2/1  "<Va>"
  Mux/1 -> LQR or Hinf?/1
  LQR or Hinf?/1 -> Demux/1
  Demux/1 -> den/1
  Demux/2 -> de/1
  vz_c/1 -> Mux4/2  "vz_c"
  Mux4/1 -> Mux3/1, Add2/1
  Va_c/1 -> Mux4/1  "Va_c"
  Mux2/1 -> Add2/2, Scope6/1
  Discrete-Time Integrator/1 -> Mux3/2
  Bus Selector/2 -> Mux2/2  "<zDot>"
  Bus Selector/5 -> Mux1/1  "<theta>"

== system formationFlyingBlockset/Fixed wing avionics/Command laws/Control laws/Trajectory law - 2/Leader following laws/Non-nested laws/LQR lateral ==
  Plant : Inport  OutDataTypeStr=Bus: StateBus
  p_lvf : Inport  Port=2
  v_lvf : Inport  Port=3
  Add3 : Sum  Inputs=-+
  Bus Selector1 : BusSelector  OutputSignals=beta_rad,omega_b_rps,quat_be
  Demux : Demux  Outputs=2
  Discrete-Time Integrator : DiscreteIntegrator  InitialConditionSetting=State (most efficient)  SampleTime=-1  ICPrevOutput=DiscIntNeverNeededParam  ICPrevScaledInput=DiscIntNeverNeededParam
  K LQR : Gain  Gain=uavsim.ap.control.lquadr.lateral.klqr  Multiplication=Matrix(K*u)
  Mux : Mux  Inputs=6
  "get p, r" : Selector  InputPortWidth=3  IndexOptions=Index vector (dialog)  Indices=[1 3]  OutputSizes=1
  get phi : Selector  InputPortWidth=3  IndexOptions=Index vector (dialog)  Indices=3  OutputSizes=1
  get vy : Selector  InputPortWidth=3  IndexOptions=Index vector (dialog)  Indices=2  OutputSizes=1
  get y : Selector  InputPortWidth=3  IndexOptions=Index vector (dialog)  Indices=2  OutputSizes=1
  quaternion to euler angles (zyx rotation) : formationFlyingBlockset/quaternion to euler  angles (zyx rotation)
  trim -1 : Constant  Value=mask_ac.beta_trim
  da : Outport
  dr : Outport  Port=2
  wires:
  Demux/2 -> dr/1
  K LQR/1 -> Demux/1
  Demux/1 -> da/1
  Mux/1 -> K LQR/1
  Discrete-Time Integrator/1 -> Mux/6
  Plant/1 -> Bus Selector1/1
  Bus Selector1/1 -> Add3/2  "<beta_rad>"
  trim -1/1 -> Add3/1
  Add3/1 -> Mux/1  "beta_lin"
  p_lvf/1 -> get y/1
  get y/1 -> Mux/3, Discrete-Time Integrator/1  "y_lin"
  Bus Selector1/2 -> "get p, r"/1  "<omega_b_rps>"
  Bus Selector1/3 -> quaternion to euler angles (zyx rotation)/1  "<quat_be>"
  quaternion to euler angles (zyx rotation)/1 -> get phi/1
  "get p, r"/1 -> Mux/4
  get phi/1 -> Mux/2
  v_lvf/1 -> get vy/1
  get vy/1 -> Mux/5

== system formationFlyingBlockset/Fixed wing avionics/Command laws/Control laws/Trajectory law - 2/Leader following laws/Non-nested laws/LQR longi ==
  y_ac : Inport
  v_lvf : Inport  Port=2
  Bus Selector : BusSelector  OutputSignals=Va,theta,q,alpha,x,z
  Demux : Demux  Outputs=2
  Discrete-Time Integrator : DiscreteIntegrator  InitialConditionSetting=State (most efficient)  SampleTime=-1  ICPrevOutput=DiscIntNeverNeededParam  ICPrevScaledInput=DiscIntNeverNeededParam
  Discrete-Time Integrator1 : DiscreteIntegrator  InitialConditionSetting=State (most efficient)  SampleTime=-1  ICPrevOutput=DiscIntNeverNeededParam  ICPrevScaledInput=DiscIntNeverNeededParam
  K LQR : Gain  Gain=uavsim.ap.control.lquadr.longi.klqr  Multiplication=Matrix(K*u)
  Mux : Mux  Inputs=8
  Scope : Scope
  get vz : Selector  InputPortWidth=3  IndexOptions=Index vector (dialog)  Indices=3  OutputSizes=1
  de : Outport
  den : Outport  Port=2
  wires:
  y_ac/1 -> Bus Selector/1
  Bus Selector/1 -> Mux/1  "<Va>"
  Bus Selector/3 -> Mux/6  "<q>"
  Bus Selector/4 -> Mux/2  "<alpha>"
  Bus Selector/5 -> Discrete-Time Integrator/1, Mux/4  "<x>"
  Bus Selector/6 -> Discrete-Time Integrator1/1, Mux/5  "<z>"
  Discrete-Time Integrator/1 -> Mux/7
  Discrete-Time Integrator1/1 -> Scope/1, Mux/8
  Mux/1 -> K LQR/1
  Demux/1 -> de/1  "de"
  K LQR/1 -> Demux/1
  Demux/2 -> den/1  "den"
  v_lvf/1 -> get vz/1
  Bus Selector/2 -> Mux/3  "<theta>"

== system formationFlyingBlockset/Fixed wing avionics/Command laws/Control laws/Trajectory law - 2/Leader following laws/Non-nested laws/LQR pos longi ==
  y_ac : Inport
  Bus Selector : BusSelector  OutputSignals=x,z,Va,zDot
  Demux : Demux  Outputs=2
  Discrete-Time Integrator : DiscreteIntegrator  InitialConditionSetting=State (most efficient)  SampleTime=-1  ICPrevOutput=DiscIntNeverNeededParam  ICPrevScaledInput=DiscIntNeverNeededParam
  Discrete-Time Integrator1 : DiscreteIntegrator  InitialConditionSetting=State (most efficient)  SampleTime=-1  ICPrevOutput=DiscIntNeverNeededParam  ICPrevScaledInput=DiscIntNeverNeededParam
  K LQR : Gain  Gain=mpc.longi.klqr_pos  Multiplication=Matrix(K*u)
  Mux2 : Mux  Inputs=6
  Va_c : Outport
  vz_c : Outport  Port=2
  wires:
  Bus Selector/1 -> Mux2/2, Discrete-Time Integrator/1  "<x>"
  y_ac/1 -> Bus Selector/1
  Bus Selector/2 -> Mux2/5, Discrete-Time Integrator1/1  "<z>"
  Bus Selector/3 -> Mux2/3  "<Va>"
  Bus Selector/4 -> Mux2/6  "<zDot>"
  Mux2/1 -> K LQR/1
  K LQR/1 -> Demux/1
  Demux/1 -> Va_c/1
  Demux/2 -> vz_c/1
  Discrete-Time Integrator/1 -> Mux2/1
  Discrete-Time Integrator1/1 -> Mux2/4

== system formationFlyingBlockset/Fixed wing avionics/Command laws/Control laws/Trajectory law - 2/Leader following laws/Non-nested laws/LQR speed longi ==
  y_ac : Inport
  Va_c : Inport  Port=2
  vz_c : Inport  Port=3
  Add : Sum  Inputs=+-
  Bus Selector : BusSelector  OutputSignals=Va,zDot,theta,q
  Demux2 : Demux  Outputs=2
  K_speed : Gain  Gain=mpc.longi.klqr_speed  Multiplication=Matrix(K*u)
  Mux2 : Mux
  Mux3 : Mux
  Scope : Scope
  nix : Ground
  de : Outport
  den : Outport  Port=2
  wires:
  Demux2/2 -> den/1  "den"
  Demux2/1 -> de/1  "de"
  K_speed/1 -> Demux2/1
  y_ac/1 -> Bus Selector/1
  Bus Selector/2 -> Scope/1, Mux3/2  "<zDot>"
  Bus Selector/1 -> Mux3/1  "<Va>"
  Bus Selector/3 -> Mux3/3  "<theta>"
  Bus Selector/4 -> Mux3/4  "<q>"
  Mux3/1 -> Add/1  "x"
  nix/1 -> Mux2/4, Mux2/3
  Mux2/1 -> Add/2
  Va_c/1 -> Mux2/1
  vz_c/1 -> Mux2/2
  Add/1 -> K_speed/1

== system formationFlyingBlockset/Fixed wing avionics/Command laws/Control laws/Trajectory law - 2/Leader following laws/Non-nested laws/Remove operating point offset longi ==
  Va : Inport  PortDimensions=1
  theta : Inport  Port=2  PortDimensions=1
  q : Inport  Port=3  PortDimensions=1
  alpha : Inport  Port=4  PortDimensions=1
  den_c : Inport  Port=5  PortDimensions=1
  - : Constant  Value=mask_ac.u_trim(4)
  Add{,1..3} (4 alike) : Sum  Inputs=-+
  Scope : Scope
  trim - : Constant  Value=mask_ac.alpha_trim
  trim state : Constant  Value=mask_ac.x_trim(5)
  trim state1 : Constant  Value=norm(mask_ac.x_trim(1:3))
  Va_lin : Outport
  theta_lin : Outport  Port=2
  q_lin : Outport  Port=3
  alpha_lin : Outport  Port=4
  den_c_lin : Outport  Port=5
  wires:
  Add3/1 -> Va_lin/1
  trim state/1 -> Add/1
  theta/1 -> Add/2
  Add/1 -> theta_lin/1
  q/1 -> q_lin/1
  alpha/1 -> Add1/2
  trim -/1 -> Add1/1
  Add1/1 -> alpha_lin/1
  den_c/1 -> Scope/1, Add2/2
  -/1 -> Add2/1
  Add2/1 -> den_c_lin/1
  Va/1 -> Add3/2
  trim state1/1 -> Add3/1

== matlab function formationFlyingBlockset/Parrot drone/MATLAB Function ==
  data: t output
function t = machinetime()
coder.extrinsic('now');
t = 0;
t = now;
end

== matlab function formationFlyingBlockset/Cularis/MATLAB Function ==
  data: t output
function t = machinetime()
coder.extrinsic('now');
t = 0;
t = now;
end

== matlab function formationFlyingBlockset/Virtual leader/MATLAB Function ==
  data: pLeader_NED_m output; vLeader_NED_mps output; t_UTC_s input
function [pLeader_NED_m, vLeader_NED_mps]  = doItNow(t_UTC_s)

%#codegen
% Holds the current trajectory to be followed:
persistent traj;
% Holds the UTC start time of the current trajectory:
persistent traj_t0_UTC_s;
% Holds the trajectory ground speed:
traj_v_mps = 15;

% The following functions use language elements that are not supported for
% code generation, they have to be replaced for implementation on the
% autopilot:
coder.extrinsic('trajectory_build');
coder.extrinsic('trajectory_smooth');
coder.extrinsic('trajectory_concatenateWaypoint');
coder.extrinsic('trajectory_getAirborne');
coder.extrinsic('trajectory_get');
coder.extrinsic('trajectory_getAcceleration');
coder.extrinsic('trajectory_display');
coder.extrinsic('trajectory_concatenateLoiterPattern');
coder.extrinsic('trajectory_gettrim');
coder.extrinsic('trajectory_getSplineLength');
coder.extrinsic('trajectory_getHorizontalCurvatureSign');
coder.extrinsic('evalin');

traj_t0_UTC_s = 0;
pLeader_NED_m = zeros(3,1);
vLeader_NED_mps = zeros(3,1);

% Load trajectory:
if isempty(traj)
    evalin('base', 'load(''benchmarkTrajectory.mat'')');
    traj = evalin('base', 'traj');
end
% Compute current position, velocity and centripetal acceleration of
% virtual leader on formation trajectory:
s = traj_v_mps * (t_UTC_s - traj_t0_UTC_s);
p = zeros(3,1);
uTangent = zeros(3,1);
[p, uTangent, ~] = trajectory_get(traj, s);

pLeader_NED_m = p;
vLeader_NED_mps = uTangent * traj_v_mps;
end

== matlab function formationFlyingBlockset/Cularis Vortex model/MATLAB Function1 ==
  data: pNED input; vNED input; CL input; qAttitude input; alpha input; beta input; p input; tsim input; VortexSig data_store_memory; Vi_bfrozen output; omegai_bfrozen output; Vi_NED output; p0_filament_left output; p0_filament_right output; dcm_ew output; debugport output
% This function writes the calling aircraft's relevant states into a global
% Simulink variable to enable Simulation of relative localization sensors,
% aerodynmaic coupling etc.
function [Vi_bfrozen, omegai_bfrozen, Vi_NED, p0_filament_left, p0_filament_right, dcm_ew, debugport] = vortex(pNED,vNED, ...
    CL, ...
    qAttitude, ...
    alpha, ...
    beta, ...
    p, ...
    tsim)
global VortexSig;
%coder.extrinsic('uavsimblockset_vortexmodel');
debugport = zeros(10,1);
ID = p.id;
VortexSig(ID).timeOfLastUpdate = tsim;
VortexSig(ID).p_NED_m = pNED;
VortexSig(ID).v_NED_mps = vNED;
VortexSig(ID).CL = CL;
VortexSig(ID).qAttitude = qAttitude;
VortexSig(ID).alpha_rad = alpha;
VortexSig(ID).beta_rad = beta;
VortexSig(ID).b_m = p.b_m;

VortexSig(ID).cbar_m = p.cbar_m;
VortexSig(ID).sweep_rad = p.sweep_rad;
VortexSig(ID).dihedral_rad = p.dihedral_rad;
VortexSig(ID).longiRefLength_m = p.longiRefLength_m;
VortexSig(ID).pNose_b_m = p.pNose_b_m;
VortexSig(ID).verticalRefLength_m = p.verticalRefLength_m;
VortexSig(ID).posFinTip_b_m = p.posFinTip_b_m;

Vi_bfrozen = zeros(3,1);
omegai_bfrozen = zeros(3,1);
Vi_NED = zeros(3,1);
p0_filament_left= zeros(3,1);
p0_filament_right = zeros(3,1);
dcm_ew = zeros(3);

[Vi_bfrozen, omegai_bfrozen, Vi_NED, p0_filament_left, p0_filament_right, dcm_ew, debugport] = ...
    uavsimblockset_vortexmodel(ID, ...
    tsim, ...
    VortexSig);
end
